simulink model "detect_color_red"  (R2016b)
settings: Solver=FixedStepAuto  StartTime=0.0  StopTime=0  RelTol=1e-3
undefined symbols (not defined in the file or in its folder): Rec, SDTV
libraries: visionconversions x4, visionsources x1
settings Model: Creator=sk  LastModifiedBy=sk
settings SolverCC: PositivePriorityOrder=on
settings DataIOCC: LoggingToFile=on
settings OptimizationCC: DefaultParameterBehavior=Inlined  MaxStackSize=64
settings DebuggingCC: ParameterTunabilityLossMsg=error
settings HardwareCC: ProdBitPerPointer=32  ProdBitPerSizeT=32  ProdBitPerPtrDiffT=32  ProdLargestAtomicInteger=Long  ProdLargestAtomicFloat=Double  ProdWordSize=32  ProdHWDeviceType=ARM Compatible->ARM Cortex
settings RTWCC: SystemTargetFile=ert.tlc  TemplateMakefile=ert_default_tmf  Description=Embedded Coder  GenerateReport=on  Toolchain=GNU GCC Raspberry Pi  IncludeHyperlinkInReport=on  LaunchReport=on  GenerateTraceInfo=on  GenerateTraceReport=on  GenerateTraceReportSl=on  GenerateTraceReportSf=on  GenerateTraceReportEml=on
settings CodeAppCC: ForceParamTrailComments=on  IgnoreCustomStorageClasses=off  OperatorAnnotations=on  SimulinkDataObjDesc=on  SFDataObjDesc=on  MATLABFcnDesc=on  InsertBlockDesc=on  MATLABSourceComments=on
settings ERTTargetCC: SupportVariableSizeSignals=on  ExtMode=on  ExtModeMexArgs='192.168.1.118' 0 17725  ERTCustomFileTemplate=example_file_process.tlc

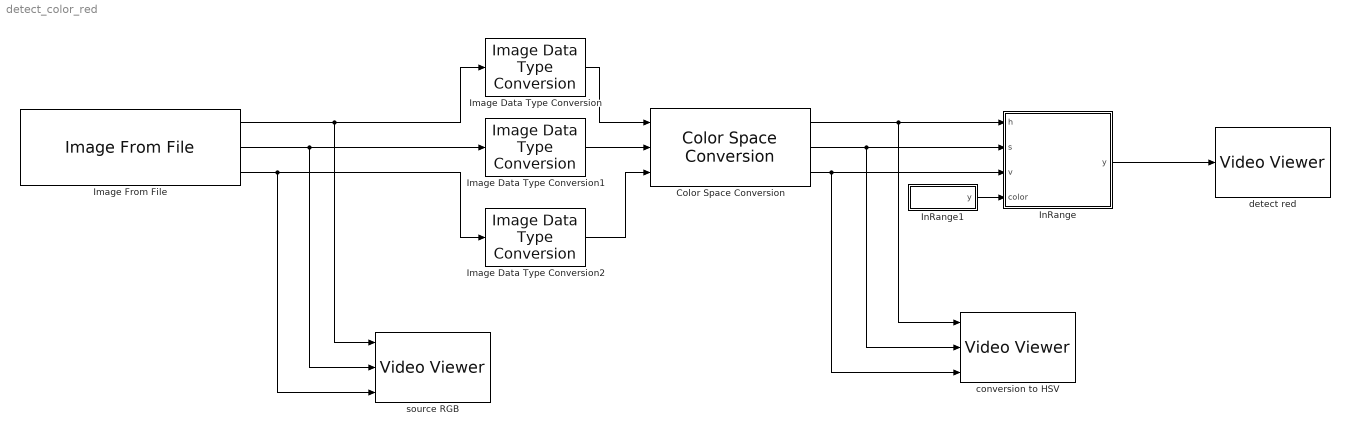
== system detect_color_red ==
  Color Space Conversion : visionconversions/Color Space  Conversion  conversion=Obsolete  conversionActive=R'G'B' to HSV  wp_str=D65  rec=Rec. 601 (SDTV)  sys=1125/60/2:1  imagePorts=Separate color signals
  Image Data Type Conversion : visionconversions/Image Data Type Conversion  outDT=single  isSigned=on  wordLen=16  numFracBits=0
  Image Data Type Conversion1 : visionconversions/Image Data Type Conversion  outDT=single  isSigned=on  wordLen=16  numFracBits=0
  Image Data Type Conversion2 : visionconversions/Image Data Type Conversion  outDT=single  isSigned=on  wordLen=16  numFracBits=0
  Image From File : visionsources/Image From File  Tag=vipblks_nd  FileName=D:\users\skconan\Workspace\MBD\Vision\images\circle.jpg  imagePorts=Separate color signals  Ts=inf  ImageDataType=Inherit from input image  Signed=on  WordLength=16  sdImageDataType=uint(8)  FractionLengthMode=User-defined  FractionLength=15  OutPortLabels=R|G|B
  InRange : MATLAB Function  TreatAsAtomicUnit=on
  InRange1 : MATLAB Function  TreatAsAtomicUnit=on
  conversion to HSV : VideoViewer  imagePorts=separate color signals  FigPos=[831 575 537 368]
  detect red : VideoViewer  FigPos=[453 594 410 300]
  source RGB : VideoViewer  imagePorts=separate color signals  FigPos=[-14 620 410 300]
  wires:
  Image From File/1 -> source RGB/1, Image Data Type Conversion/1
  Color Space Conversion/1 -> InRange/1(h), conversion to HSV/1
  Image Data Type Conversion/1 -> Color Space Conversion/1
  Image From File/2 -> source RGB/2, Image Data Type Conversion1/1
  Image From File/3 -> source RGB/3, Image Data Type Conversion2/1
  Image Data Type Conversion1/1 -> Color Space Conversion/2
  Image Data Type Conversion2/1 -> Color Space Conversion/3
  Color Space Conversion/2 -> InRange/2(s), conversion to HSV/2
  Color Space Conversion/3 -> InRange/3(v), conversion to HSV/3
  InRange/1(y) -> detect red/1
  InRange1/1(y) -> InRange/4(color)

== matlab function detect_color_red/InRange1 ==
  data: y output
% author : Supakit Kriangkhajorn
% skconan
function y = color()
    y = uint8('r');

== matlab function detect_color_red/InRange ==
  data: h input; y output; s input; v input; color input
% author : Supakit Kriangkhajorn
% skconan
function y = inRange(h,s,v,color)
    lower0 = [0,0,0];
    upper0 = [1,1,1];
    
    lower1 = [0,0,0];
    upper1 = [1,1,1];
    switch color
        case uint8('o')
            lower0 = [0/180,0,0];
            upper0  = [22/180,1,1];
        case uint8('y')
            lower0 = [23/180,0,0];
            upper0  = [38/180,1,1];
        case uint8('g')
            lower0 = [39/180,0,0];
            upper0  = [75/180,1,1];
        case uint8('b')
            lower0 = [76/180,0,0];
            upper0  = [130/180,1,1];
        case uint8('v')
            lower0 = [131/180,0,0];
            upper0  = [160/180,1,1];
        case uint8('r')
            lower0 = [0.88,0.5,0.5];
            upper0 = [1,1,1];
            
            lower1 = [0,0.5,0.5];
            upper1 = [0.23,1,1];
    end
  
    h0 = h >= lower0(1) & h <= upper0(1);
    s0 = s >= lower0(2) & s <= upper0(2);
    v0 = v >= lower0(3) & v <= upper0(3);
    
    h1 = h >= lower1(1) & h <= upper1(1);
    s1 = s >= lower1(2) & s <= upper1(2);
    v1 = v >= lower1(3) & v <= upper1(3);
    
    im1 = h0 & s0 & v0;
    im2 = h1 & s1 & v1;

    result = im1 | im2;
    
y = uint8(result)*255;
